simulink model "MECROKA_TWR_BLDC_02_controller_v3_1_work1"  (R2024a)
settings: Solver=FixedStepAuto  StartTime=0.0  StopTime=50  RelTol=1e-3  EnableMultiTasking=on
model workspace (MATLAB code in the model file):
  | num_pol_pairs = 7;
  | res_period = 5000;
  | res_pwm   = 2^8;
  | 
  | whl.rad = 0.045;
  | axle.length=0.18;
undefined symbols (not defined in the file): DiscIntNeverNeededParam
libraries: MecRoKa_SFunction_Library x16, simulink x3, slpidlib x1
settings Model: ExtModeTrigDuration=2  Creator=Bitsch  LastModifiedBy=Ishant
settings SolverCC: AlgebraicLoopSolver=TrustRegion  AutoInsertRateTranBlk=on
settings OptimizationCC: EnhancedBackFolding=on  PassReuseOutputArgsAs=Individual arguments  ZeroExternalMemoryAtStartup=off  ZeroInternalMemoryAtStartup=off  MaxStackSize=64  OptimizeBlockOrder=speed  DifferentSizesBufferReuse=on  EfficientTunableParamExpr=on
settings DebuggingCC: ParameterPrecisionLossMsg=none  ParameterTunabilityLossMsg=error  UnconnectedInputMsg=warning  UnconnectedOutputMsg=warning  UnconnectedLineMsg=warning
settings HardwareCC: ProdBitPerPointer=32  ProdBitPerSizeT=32  ProdBitPerPtrDiffT=32  ProdLargestAtomicInteger=Long  ProdLargestAtomicFloat=Double  ProdWordSize=32  ProdHWDeviceType=ARM Compatible->ARM Cortex
settings ModelReferenceCC: EnableRefExpFcnMdlSchedulingChecks=on
settings SFSimCC: MATLABDynamicMemAlloc=off
settings RTWCC: Description=Embedded Coder  SystemTargetFile=ert.tlc  HardwareBoard=Arduino MKR WiFi 1010  TemplateMakefile=ert_default_tmf  Toolchain=Arduino ARM  BuildConfiguration=Faster Runs  GPUComputeCapability=3.5
settings CodeAppCC: ForceParamTrailComments=on  IgnoreCustomStorageClasses=off  MaxIdLength=255  OperatorAnnotations=on  SimulinkDataObjDesc=on  SFDataObjDesc=on  InsertBlockDesc=on
settings ERTTargetCC: SupportContinuousTime=on  SupportVariableSizeSignals=on  ExtModeStaticAllocSize=8192

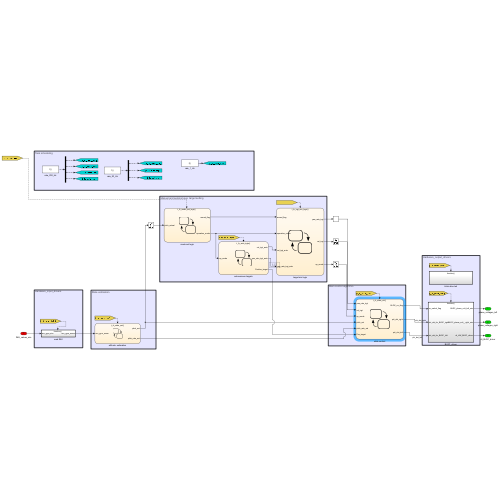
[thumbnail: Simulink's stored preview of the top-level diagram]
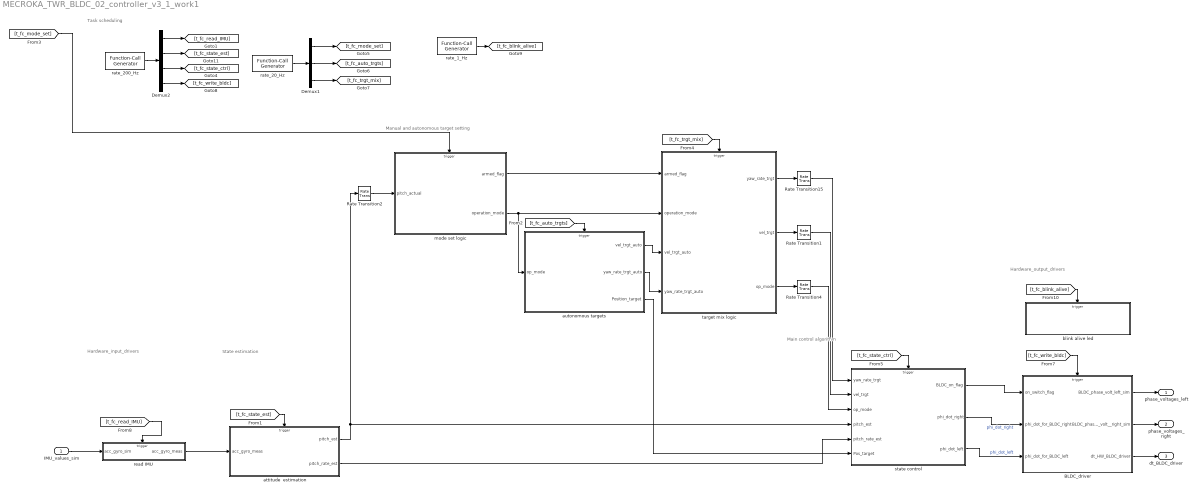
== system MECROKA_TWR_BLDC_02_controller_v3_1_work1 ==
  note: Hardware_output_drivers
  note: Main control algorithm
  note: State estimation
  note: Task scheduling
  note: Manual and autonomous target setting
  note: Hardware_input_drivers
  IMU_values_sim : Inport  OutDataTypeStr=int32  PortDimensions=6
  BLDC_driver : Subsystem  TreatAsAtomicUnit=on
  Demux1 : Demux  Outputs=3
  Demux2 : Demux
  Rate Transition{1..2,4,15} (4 alike) : RateTransition  OutPortSampleTimeOpt=Inherit  OutPortSampleTime=0.01
  attitude  estimation : Stateflow chart  TreatAsAtomicUnit=on
  autonomous targets : Stateflow chart  TreatAsAtomicUnit=on
  blink alive led : Subsystem  TreatAsAtomicUnit=on
  mode set logic : Stateflow chart  TreatAsAtomicUnit=on
  rate_1_Hz : simulink/Ports & Subsystems/Function-Call Generator  sample_time=0.5  numberOfIterations=1  DisallowWideOutput=off
  rate_200_Hz : simulink/Ports & Subsystems/Function-Call Generator  sample_time=0.005  numberOfIterations=1  DisallowWideOutput=off
  rate_20_Hz : simulink/Ports & Subsystems/Function-Call Generator  sample_time=0.05  numberOfIterations=1  DisallowWideOutput=off
  read IMU : Subsystem  TreatAsAtomicUnit=on
  state control : Stateflow chart  TreatAsAtomicUnit=on
  target mix logic : Stateflow chart  TreatAsAtomicUnit=on
  phase_voltages_left : Outport
  phase_voltages_right : Outport  Port=2
  dt_BLDC_driver : Outport  Port=3
  wires:
  autonomous targets/1(vel_trgt_auto) -> target mix logic/3(vel_trgt_auto)
  attitude  estimation/1(pitch_est) -> Rate Transition2/1, state control/4(pitch_est)
  state control/2(phi_dot_right) -> BLDC_driver/2(phi_dot_for_BLDC_right)  "phi_dot_right"
  [t_fc_trgt_mix] -> target mix logic/Trigger
  [t_fc_read_IMU] -> read IMU/Trigger
  [t_fc_state_est] -> attitude  estimation/Trigger
  Demux2/3 -> [t_fc_state_ctrl]
  Demux1/2 -> [t_fc_auto_trgts]
  Demux2/4 -> [t_fc_write_bldc]
  target mix logic/3(op_mode) -> Rate Transition4/1
  Rate Transition1/1 -> state control/2(vel_trgt)
  Demux2/1 -> [t_fc_read_IMU]
  mode set logic/1(armed_flag) -> target mix logic/1(armed_flag)
  Rate Transition15/1 -> state control/1(yaw_rate_trgt)
  Demux2/2 -> [t_fc_state_est]
  attitude  estimation/2(pitch_rate_est) -> state control/5(pitch_rate_est)
  mode set logic/2(operation_mode) -> autonomous targets/1(op_mode), target mix logic/2(operation_mode)
  IMU_values_sim/1 -> read IMU/1(acc_gyro_sim)
  [t_fc_mode_set] -> mode set logic/Trigger
  rate_200_Hz/1 -> Demux2/1
  state control/1(BLDC_on_flag) -> BLDC_driver/1(on_switch_flag)
  Rate Transition2/1 -> mode set logic/1(pitch_actual)
  [t_fc_blink_alive] -> blink alive led/Trigger
  BLDC_driver/1(BLDC_phase_volt_left_sim) -> phase_voltages_left/1
  [t_fc_auto_trgts] -> autonomous targets/Trigger
  Rate Transition4/1 -> state control/3(op_mode)
  autonomous targets/2(yaw_rate_trgt_auto) -> target mix logic/4(yaw_rate_trgt_auto)
  BLDC_driver/2(BLDC_phase_volt__right_sim) -> phase_voltages_right/1
  Demux1/3 -> [t_fc_trgt_mix]
  [t_fc_write_bldc] -> BLDC_driver/Trigger
  Demux1/1 -> [t_fc_mode_set]
  state control/3(phi_dot_left) -> BLDC_driver/3(phi_dot_for_BLDC_left)  "phi_dot_left"
  rate_20_Hz/1 -> Demux1/1
  read IMU/1(acc_gyro_meas) -> attitude  estimation/1(acc_gyro_meas)
  [t_fc_state_ctrl] -> state control/Trigger
  rate_1_Hz/1 -> [t_fc_blink_alive]
  target mix logic/1(yaw_rate_trgt) -> Rate Transition15/1
  target mix logic/2(vel_trgt) -> Rate Transition1/1
  BLDC_driver/3(dt_HW_BLDC_driver) -> dt_BLDC_driver/1
  autonomous targets/3(Position_target) -> state control/6(Pos_target)

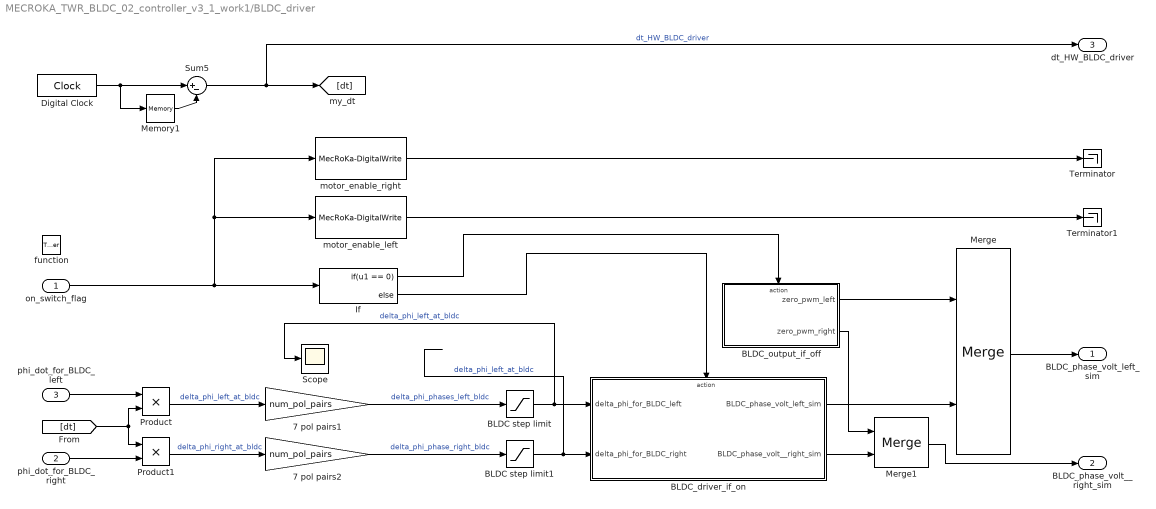
== system MECROKA_TWR_BLDC_02_controller_v3_1_work1/BLDC_driver ==
  on_switch_flag : Inport  OutDataTypeStr=boolean  PortDimensions=1
  phi_dot_for_BLDC_right : Inport  Port=2  OutDataTypeStr=double  PortDimensions=1
  phi_dot_for_BLDC_left : Inport  Port=3  OutDataTypeStr=double  PortDimensions=1
  function : TriggerPort  TriggerType=function-call  VariantControl=(inherit)
  7 pol pairs1 : Gain  Gain=num_pol_pairs
  7 pol pairs2 : Gain  Gain=num_pol_pairs
  BLDC step limit : Saturate  UpperLimit=2  LowerLimit=-2
  BLDC step limit1 : Saturate  UpperLimit=2  LowerLimit=-2
  BLDC_driver_if_on : Subsystem  TreatAsAtomicUnit=on
  BLDC_output_if_off : Subsystem  TreatAsAtomicUnit=on
  Digital Clock : DigitalClock  SampleTime=-1
  If : If  IfExpression=u1 == 0
  Memory1 : Memory  InitialCondition=-0.005  InheritSampleTime=on  LinearizeAsDelay=on
  Merge : Merge
  Merge1 : Merge
  Product : Product
  Product1 : Product
  Scope : Scope
  Sum5 : Sum  Inputs=|+-
  Terminator : Terminator
  Terminator1 : Terminator
  motor_enable_left : MecRoKa_SFunction_Library/Arduino-Blocks/Arduino-Library/MecRoKa-DigitalWrite  pinNumber=7
      settings: SourceProductName=MecRoKa_SFunction-Library
  motor_enable_right : MecRoKa_SFunction_Library/Arduino-Blocks/Arduino-Library/MecRoKa-DigitalWrite  pinNumber=6
      settings: SourceProductName=MecRoKa_SFunction-Library
  BLDC_phase_volt_left_sim : Outport  OutDataTypeStr=uint16  PortDimensions=3
  BLDC_phase_volt__right_sim : Outport  Port=2  OutDataTypeStr=uint16  PortDimensions=3
  dt_HW_BLDC_driver : Outport  Port=3
  wires:
  phi_dot_for_BLDC_right/1 -> Product1/2
  on_switch_flag/1 -> motor_enable_left/1, motor_enable_right/1, If/1
  BLDC_output_if_off/1(zero_pwm_left) -> Merge/1
  Merge/1 -> BLDC_phase_volt_left_sim/1
  If/1 -> BLDC_output_if_off/Action
  Merge1/1 -> BLDC_phase_volt__right_sim/1
  BLDC_driver_if_on/1(BLDC_phase_volt_left_sim) -> Merge/2
  If/2 -> BLDC_driver_if_on/Action
  BLDC_driver_if_on/2(BLDC_phase_volt__right_sim) -> Merge1/2
  BLDC_output_if_off/2(zero_pwm_right) -> Merge1/1
  phi_dot_for_BLDC_left/1 -> Product/1
  7 pol pairs2/1 -> BLDC step limit1/1  "delta_phi_phase_right_bldc"
  7 pol pairs1/1 -> BLDC step limit/1  "delta_phi_phases_left_bldc"
  Digital Clock/1 -> Memory1/1, Sum5/1
  Sum5/1 -> dt_HW_BLDC_driver/1, [dt]  "dt_HW_BLDC_driver"
  Memory1/1 -> Sum5/2
  [dt] -> Product1/1, Product/2
  Product/1 -> 7 pol pairs1/1  "delta_phi_left_at_bldc"
  Product1/1 -> 7 pol pairs2/1  "delta_phi_right_at_bldc"
  BLDC step limit/1 -> Scope/1, BLDC_driver_if_on/1(delta_phi_for_BLDC_left)  "delta_phi_left_at_bldc"
  BLDC step limit1/1 -> BLDC_driver_if_on/2(delta_phi_for_BLDC_right)  "delta_phi_left_at_bldc"
  motor_enable_right/1 -> Terminator/1
  motor_enable_left/1 -> Terminator1/1

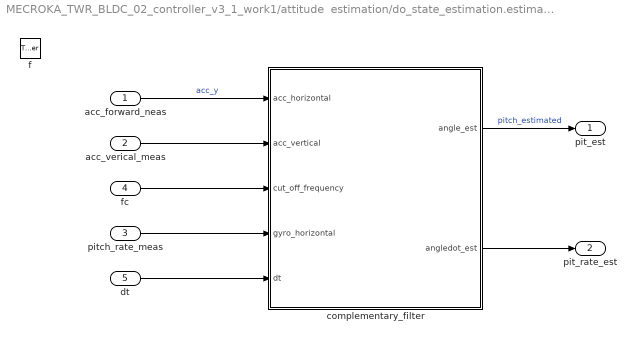
== system MECROKA_TWR_BLDC_02_controller_v3_1_work1/attitude  estimation/do_state_estimation.estimate_angulars_graph ==
  acc_forward_neas : Inport  OutDataTypeStr=double  PortDimensions=1
  acc_verical_meas : Inport  Port=2  OutDataTypeStr=double  PortDimensions=1
  pitch_rate_meas : Inport  Port=3  OutDataTypeStr=double  PortDimensions=1  LockScale=on
  fc : Inport  Port=4  OutDataTypeStr=double  PortDimensions=1
  dt : Inport  Port=5  OutDataTypeStr=double  PortDimensions=1
  f : TriggerPort  TriggerType=function-call  VariantControl=(inherit)
      settings: CopyFcn=Stateflow.SLINSF.SimulinkMan.removeBlockPreDeleteFcn  PreDeleteFcn=Stateflow.SLINSF.SimulinkMan.unsafePredeleteFcn
  complementary_filter : Subsystem
  pit_est : Outport  OutDataTypeStr=double
  pit_rate_est : Outport  Port=2  OutDataTypeStr=double
  wires:
  acc_verical_meas/1 -> complementary_filter/2(acc_vertical)
  pitch_rate_meas/1 -> complementary_filter/4(gyro_horizontal)
  acc_forward_neas/1 -> complementary_filter/1(acc_horizontal)  "acc_y"
  fc/1 -> complementary_filter/3(cut_off_frequency)
  complementary_filter/2(angledot_est) -> pit_rate_est/1
  complementary_filter/1(angle_est) -> pit_est/1  "pitch_estimated"
  dt/1 -> complementary_filter/5(dt)

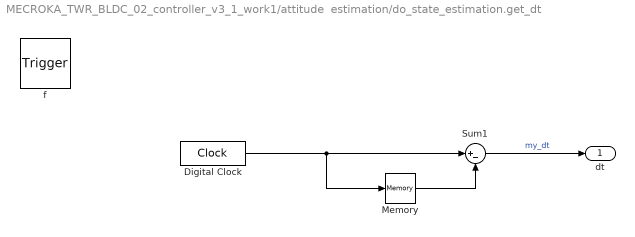
== system MECROKA_TWR_BLDC_02_controller_v3_1_work1/attitude  estimation/do_state_estimation.get_dt ==
  f : TriggerPort  TriggerType=function-call  VariantControl=(inherit)
      settings: CopyFcn=Stateflow.SLINSF.SimulinkMan.removeBlockPreDeleteFcn  PreDeleteFcn=Stateflow.SLINSF.SimulinkMan.unsafePredeleteFcn
  Digital Clock : DigitalClock  SampleTime=-1
  Memory : Memory  InitialCondition=-0.005  InheritSampleTime=on  LinearizeAsDelay=on
  Sum1 : Sum  Inputs=|+-
  dt : Outport
  wires:
  Sum1/1 -> dt/1  "my_dt"
  Digital Clock/1 -> Memory/1, Sum1/1
  Memory/1 -> Sum1/2

== system MECROKA_TWR_BLDC_02_controller_v3_1_work1/blink alive led ==
  function : TriggerPort  TriggerType=function-call  VariantControl=(inherit)
  MecRoKa-TogglePin : MecRoKa_SFunction_Library/Arduino-Blocks/Arduino-Library/MecRoKa-TogglePin  pinNumber=13
      settings: SourceProductName=MecRoKa_SFunction-Library

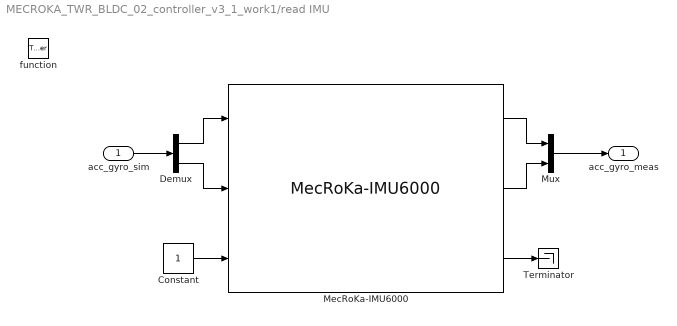
== system MECROKA_TWR_BLDC_02_controller_v3_1_work1/read IMU ==
  acc_gyro_sim : Inport  OutDataTypeStr=int32  PortDimensions=6
  function : TriggerPort  TriggerType=function-call  VariantControl=(inherit)
  Constant : Constant  OutDataTypeStr=int32
  Demux : Demux  Outputs=2
  MecRoKa-IMU6000 : MecRoKa_SFunction_Library/Arduino-Blocks/Sensor-Library/MecRoKa-IMU6000  selectWire=0
      settings: SourceProductName=MecRoKa_SFunction-Library
  Mux : Mux  Inputs=2
  Terminator : Terminator
  acc_gyro_meas : Outport  OutDataTypeStr=int32  PortDimensions=6
  wires:
  acc_gyro_sim/1 -> Demux/1
  Mux/1 -> acc_gyro_meas/1
  Demux/1 -> MecRoKa-IMU6000/1
  Demux/2 -> MecRoKa-IMU6000/2
  MecRoKa-IMU6000/1 -> Mux/1
  MecRoKa-IMU6000/2 -> Mux/2
  MecRoKa-IMU6000/3 -> Terminator/1
  Constant/1 -> MecRoKa-IMU6000/3

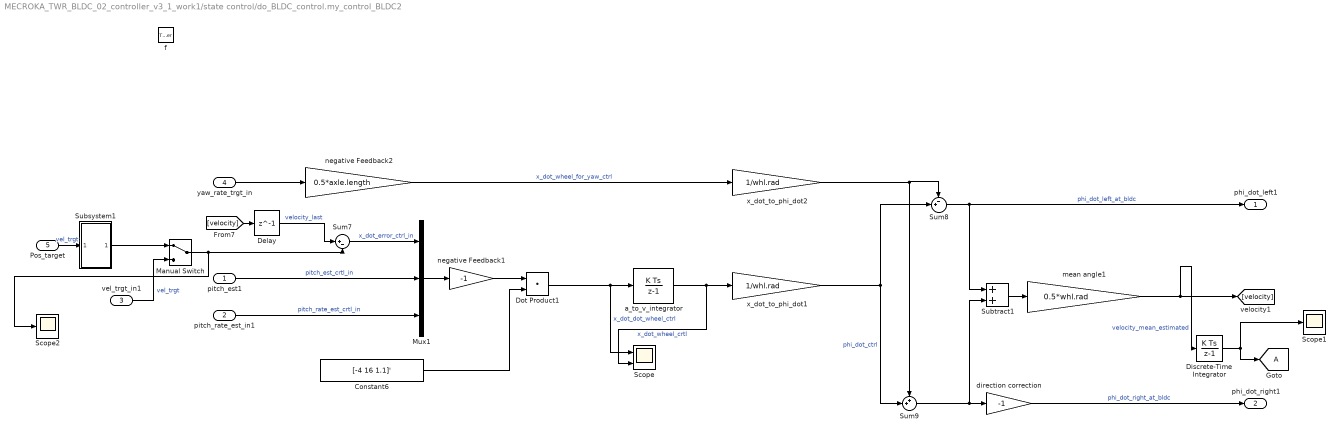
== system MECROKA_TWR_BLDC_02_controller_v3_1_work1/state control/do_BLDC_control.my_control_BLDC2 ==
  pitch_est1 : Inport  OutDataTypeStr=double  PortDimensions=1
  pitch_rate_est_in1 : Inport  Port=2  OutDataTypeStr=double  PortDimensions=1
  vel_trgt_in1 : Inport  Port=3  OutDataTypeStr=double  PortDimensions=1
  yaw_rate_trgt_in : Inport  Port=4  OutDataTypeStr=double  PortDimensions=1
  Pos_target : Inport  Port=5  OutDataTypeStr=double  PortDimensions=1
  f : TriggerPort  TriggerType=function-call  VariantControl=(inherit)
      settings: CopyFcn=Stateflow.SLINSF.SimulinkMan.removeBlockPreDeleteFcn  PreDeleteFcn=Stateflow.SLINSF.SimulinkMan.unsafePredeleteFcn
  Constant6 : Constant  Value=[-4 16 1.1]'  OutDataTypeStr=double
  Delay : Delay  DelayLength=1  InitialCondition=0
  Discrete-Time Integrator : DiscreteIntegrator  SampleTime=-1  ICPrevOutput=DiscIntNeverNeededParam  ICPrevScaledInput=DiscIntNeverNeededParam
  Dot Product1 : DotProduct  OutDataTypeStr=Inherit: Inherit via internal rule
  Goto : Goto  TagVisibility=global
  Manual Switch : ManualSwitch
  Mux1 : Mux  Inputs=3
  Scope : Scope  NumInputPorts=2
  Scope1 : Scope
  Scope2 : Scope
  Subsystem1 : Subsystem
  Subtract1 : Sum
  Sum7 : Sum  Inputs=|+-
  Sum8 : Sum  Inputs=-+|
  Sum9 : Sum  Inputs=++|
  a_to_v_integrator : DiscreteIntegrator  SampleTime=-1  LimitOutput=on  UpperSaturationLimit=2  LowerSaturationLimit=-5  ICPrevOutput=DiscIntNeverNeededParam  ICPrevScaledInput=DiscIntNeverNeededParam
  direction correction : Gain  Gain=-1
  mean angle1 : Gain  Gain=0.5*whl.rad  OutDataTypeStr=double
  negative Feedback1 : Gain  Gain=-1
  negative Feedback2 : Gain  Gain=0.5*axle.length
  x_dot_to_phi_dot1 : Gain  Gain=1/whl.rad
  x_dot_to_phi_dot2 : Gain  Gain=1/whl.rad
  phi_dot_left1 : Outport  OutDataTypeStr=double  PortDimensions=1
  phi_dot_right1 : Outport  Port=2  OutDataTypeStr=double  PortDimensions=1
  wires:
  Mux1/1 -> negative Feedback1/1
  negative Feedback1/1 -> Dot Product1/1
  Sum7/1 -> Mux1/1  "x_dot_error_ctrl_in"
  Constant6/1 -> Dot Product1/2
  yaw_rate_trgt_in/1 -> negative Feedback2/1
  x_dot_to_phi_dot2/1 -> Sum9/1, Sum8/1
  [velocity] -> Delay/1
  vel_trgt_in1/1 -> Manual Switch/2  "vel_trgt"
  pitch_est1/1 -> Mux1/2  "pitch_est_crtl_in"
  pitch_rate_est_in1/1 -> Mux1/3  "pitch_rate_est_crtl_in"
  Dot Product1/1 -> Scope/1, a_to_v_integrator/1  "x_dot_dot_wheel_ctrl"
  x_dot_to_phi_dot1/1 -> Sum9/2, Sum8/2  "phi_dot_ctrl"
  Sum9/1 -> Subtract1/2, direction correction/1
  Subtract1/1 -> mean angle1/1
  Delay/1 -> Sum7/1  "velocity_last"
  Sum8/1 -> Subtract1/1, phi_dot_left1/1  "phi_dot_left_at_bldc"
  direction correction/1 -> phi_dot_right1/1  "phi_dot_right_at_bldc"
  a_to_v_integrator/1 -> Scope/2, x_dot_to_phi_dot1/1  "x_dot_wheel_crtl"
  negative Feedback2/1 -> x_dot_to_phi_dot2/1  "x_dot_wheel_for_yaw_ctrl"
  mean angle1/1 -> Discrete-Time Integrator/1, [velocity]  "velocity_mean_estimated"
  Discrete-Time Integrator/1 -> Goto/1, Scope1/1
  Subsystem1/1(Output) -> Manual Switch/1
  Manual Switch/1 -> Scope2/1, Sum7/2
  Pos_target/1 -> Subsystem1/1(Input)  "vel_trgt"

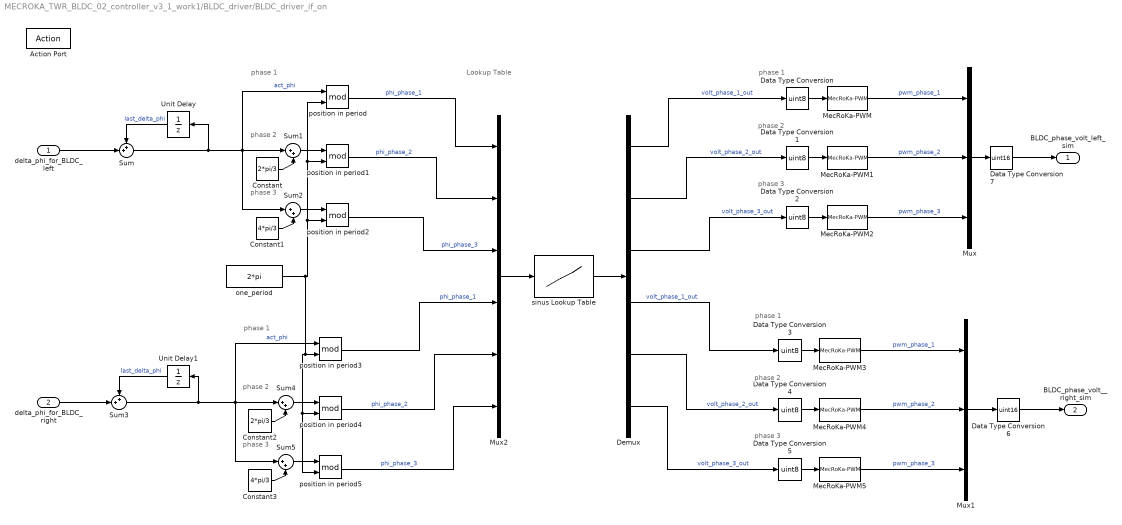
== system MECROKA_TWR_BLDC_02_controller_v3_1_work1/BLDC_driver/BLDC_driver_if_on ==
  note: Lookup Table
  note: phase 3
  note: phase 2
  note: phase 1
  note: phase 3
  note: phase 2
  note: phase 1
  note: phase 1
  note: phase 2
  note: phase 3
  note: phase 3
  note: phase 1
  note: phase 2
  delta_phi_for_BLDC_left : Inport  OutDataTypeStr=double  PortDimensions=1
  delta_phi_for_BLDC_right : Inport  Port=2  OutDataTypeStr=double  PortDimensions=1
  Action Port : ActionPort  ActionPortLabel=else
  Constant : Constant  Value=2*pi/3
  Constant1 : Constant  Value=4*pi/3
  Constant2 : Constant  Value=2*pi/3
  Constant3 : Constant  Value=4*pi/3
  Data Type Conversion{,1..5} (6 alike) : DataTypeConversion  OutDataTypeStr=uint8  SaturateOnIntegerOverflow=off  RndMeth=Floor
  Data Type Conversion6 : DataTypeConversion  OutDataTypeStr=uint16  SaturateOnIntegerOverflow=off  RndMeth=Floor
  Data Type Conversion7 : DataTypeConversion  OutDataTypeStr=uint16  SaturateOnIntegerOverflow=off  RndMeth=Floor
  Demux : Demux  Outputs=6
  MecRoKa-PWM : MecRoKa_SFunction_Library/Arduino-Blocks/Arduino-Library/MecRoKa-PWM  pinNumber=0
      settings: SourceProductName=MecRoKa_SFunction-Library
  MecRoKa-PWM1 : MecRoKa_SFunction_Library/Arduino-Blocks/Arduino-Library/MecRoKa-PWM  pinNumber=1
      settings: SourceProductName=MecRoKa_SFunction-Library
  MecRoKa-PWM2 : MecRoKa_SFunction_Library/Arduino-Blocks/Arduino-Library/MecRoKa-PWM  pinNumber=2
      settings: SourceProductName=MecRoKa_SFunction-Library
  MecRoKa-PWM3 : MecRoKa_SFunction_Library/Arduino-Blocks/Arduino-Library/MecRoKa-PWM  pinNumber=3
      settings: SourceProductName=MecRoKa_SFunction-Library
  MecRoKa-PWM4 : MecRoKa_SFunction_Library/Arduino-Blocks/Arduino-Library/MecRoKa-PWM  pinNumber=4
      settings: SourceProductName=MecRoKa_SFunction-Library
  MecRoKa-PWM5 : MecRoKa_SFunction_Library/Arduino-Blocks/Arduino-Library/MecRoKa-PWM  pinNumber=5
      settings: SourceProductName=MecRoKa_SFunction-Library
  Mux : Mux  Inputs=3
  Mux1 : Mux  Inputs=3
  Mux2 : Mux  Inputs=6
  Sum : Sum  Inputs=++|
  Sum{1..2,4..5} (4 alike) : Sum  Inputs=|++
  Sum3 : Sum  Inputs=++|
  Unit Delay : UnitDelay  SampleTime=-1  HasFrameUpgradeWarning=on
  Unit Delay1 : UnitDelay  SampleTime=-1  HasFrameUpgradeWarning=on
  one_period : Constant  Value=2*pi
  position in period{,1..5} (6 alike) : Math  Operator=mod  SignedPower=on
  sinus Lookup Table : Lookup_n-D  NumberOfTableDimensions=1  BreakpointsSpecification=Even spacing  BreakpointsForDimension1=[0:0.25:2*pi]  BreakpointsForDimension2=[0:0.25:2*pi]  BreakpointsForDimension3=[0:0.25:2*pi]  BreakpointsForDimension1FirstPoint=0  BreakpointsForDimension1Spacing=2*pi/res_period  BreakpointsForDimension2Spacing=0.25  BreakpointsForDimension3Spacing=0.25  BeginIndexSearchUsingPreviousIndexResult=on  Table=(res_pwm/2-1)*sin([0:2*pi/res_period:2*pi])+(res_pwm/2-1)  InterpMethod=Nearest  ExtrapMethod=Cubic spline  InternalRulePriority=Speed  OutDataTypeStr=uint16  RndMeth=Simplest
  BLDC_phase_volt_left_sim : Outport  OutDataTypeStr=uint16  PortDimensions=3
  BLDC_phase_volt__right_sim : Outport  Port=2  OutDataTypeStr=uint16  PortDimensions=3
  wires:
  Demux/1 -> Data Type Conversion/1  "volt_phase_1_out"
  Unit Delay/1 -> Sum/1  "last_delta_phi"
  Sum/1 -> position in period/1, Sum2/1, Sum1/1, Unit Delay/1  "act_phi"
  Sum1/1 -> position in period1/1
  Sum2/1 -> position in period2/1
  Constant/1 -> Sum1/2
  position in period1/1 -> Mux2/2  "phi_phase_2"
  position in period2/1 -> Mux2/3  "phi_phase_3"
  Demux/2 -> Data Type Conversion1/1  "volt_phase_2_out"
  Demux/3 -> Data Type Conversion2/1  "volt_phase_3_out"
  Constant1/1 -> Sum2/2
  position in period/1 -> Mux2/1  "phi_phase_1"
  Mux/1 -> Data Type Conversion7/1
  Data Type Conversion/1 -> MecRoKa-PWM/1
  Data Type Conversion1/1 -> MecRoKa-PWM1/1
  Data Type Conversion2/1 -> MecRoKa-PWM2/1
  MecRoKa-PWM/1 -> Mux/1  "pwm_phase_1"
  MecRoKa-PWM1/1 -> Mux/2  "pwm_phase_2"
  MecRoKa-PWM2/1 -> Mux/3  "pwm_phase_3"
  delta_phi_for_BLDC_left/1 -> Sum/2
  one_period/1 -> position in period5/2, position in period4/2, position in period3/2, position in period/2, position in period1/2, position in period2/2
  Unit Delay1/1 -> Sum3/1  "last_delta_phi"
  Sum3/1 -> position in period3/1, Sum5/1, Sum4/1, Unit Delay1/1  "act_phi"
  Sum4/1 -> position in period4/1
  Sum5/1 -> position in period5/1
  Constant2/1 -> Sum4/2
  position in period4/1 -> Mux2/5  "phi_phase_2"
  position in period5/1 -> Mux2/6  "phi_phase_3"
  Constant3/1 -> Sum5/2
  position in period3/1 -> Mux2/4  "phi_phase_1"
  Mux1/1 -> Data Type Conversion6/1
  Data Type Conversion3/1 -> MecRoKa-PWM3/1
  Data Type Conversion4/1 -> MecRoKa-PWM4/1
  Data Type Conversion5/1 -> MecRoKa-PWM5/1
  MecRoKa-PWM3/1 -> Mux1/1  "pwm_phase_1"
  MecRoKa-PWM4/1 -> Mux1/2  "pwm_phase_2"
  MecRoKa-PWM5/1 -> Mux1/3  "pwm_phase_3"
  Demux/4 -> Data Type Conversion3/1  "volt_phase_1_out"
  Demux/5 -> Data Type Conversion4/1  "volt_phase_2_out"
  Demux/6 -> Data Type Conversion5/1  "volt_phase_3_out"
  delta_phi_for_BLDC_right/1 -> Sum3/2
  Data Type Conversion7/1 -> BLDC_phase_volt_left_sim/1
  Data Type Conversion6/1 -> BLDC_phase_volt__right_sim/1
  Mux2/1 -> sinus Lookup Table/1
  sinus Lookup Table/1 -> Demux/1

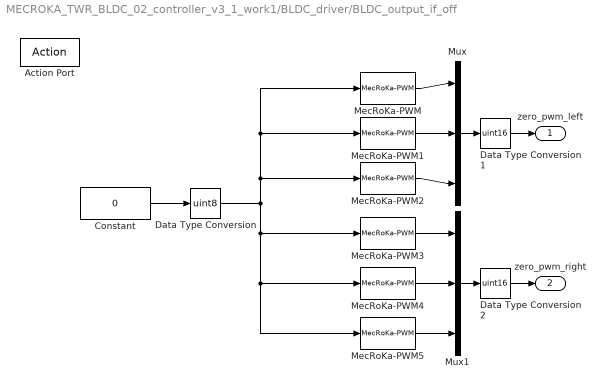
== system MECROKA_TWR_BLDC_02_controller_v3_1_work1/BLDC_driver/BLDC_output_if_off ==
  Action Port : ActionPort  ActionPortLabel=if(u1 == 0)
  Constant : Constant  Value=0  OutDataTypeStr=uint16
  Data Type Conversion : DataTypeConversion  OutDataTypeStr=uint8  SaturateOnIntegerOverflow=off  RndMeth=Floor
  Data Type Conversion1 : DataTypeConversion  OutDataTypeStr=uint16  SaturateOnIntegerOverflow=off  RndMeth=Floor
  Data Type Conversion2 : DataTypeConversion  OutDataTypeStr=uint16  SaturateOnIntegerOverflow=off  RndMeth=Floor
  MecRoKa-PWM : MecRoKa_SFunction_Library/Arduino-Blocks/Arduino-Library/MecRoKa-PWM  pinNumber=0
      settings: SourceProductName=MecRoKa_SFunction-Library
  MecRoKa-PWM1 : MecRoKa_SFunction_Library/Arduino-Blocks/Arduino-Library/MecRoKa-PWM  pinNumber=1
      settings: SourceProductName=MecRoKa_SFunction-Library
  MecRoKa-PWM2 : MecRoKa_SFunction_Library/Arduino-Blocks/Arduino-Library/MecRoKa-PWM  pinNumber=2
      settings: SourceProductName=MecRoKa_SFunction-Library
  MecRoKa-PWM3 : MecRoKa_SFunction_Library/Arduino-Blocks/Arduino-Library/MecRoKa-PWM  pinNumber=3
      settings: SourceProductName=MecRoKa_SFunction-Library
  MecRoKa-PWM4 : MecRoKa_SFunction_Library/Arduino-Blocks/Arduino-Library/MecRoKa-PWM  pinNumber=4
      settings: SourceProductName=MecRoKa_SFunction-Library
  MecRoKa-PWM5 : MecRoKa_SFunction_Library/Arduino-Blocks/Arduino-Library/MecRoKa-PWM  pinNumber=5
      settings: SourceProductName=MecRoKa_SFunction-Library
  Mux : Mux  Inputs=3
  Mux1 : Mux  Inputs=3
  zero_pwm_left : Outport
  zero_pwm_right : Outport  Port=2
  wires:
  Constant/1 -> Data Type Conversion/1
  Data Type Conversion/1 -> MecRoKa-PWM5/1, MecRoKa-PWM4/1, MecRoKa-PWM3/1, MecRoKa-PWM1/1, MecRoKa-PWM/1, MecRoKa-PWM2/1
  MecRoKa-PWM/1 -> Mux/1
  MecRoKa-PWM1/1 -> Mux/2
  MecRoKa-PWM2/1 -> Mux/3
  MecRoKa-PWM3/1 -> Mux1/1
  MecRoKa-PWM4/1 -> Mux1/2
  MecRoKa-PWM5/1 -> Mux1/3
  Mux1/1 -> Data Type Conversion2/1
  Mux/1 -> Data Type Conversion1/1
  Data Type Conversion1/1 -> zero_pwm_left/1
  Data Type Conversion2/1 -> zero_pwm_right/1

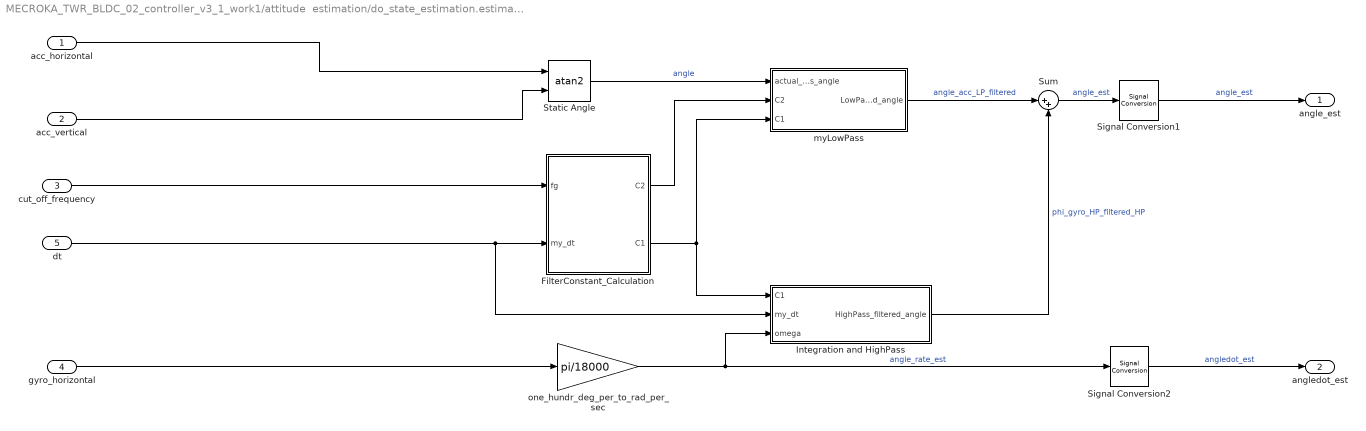
== system MECROKA_TWR_BLDC_02_controller_v3_1_work1/attitude  estimation/do_state_estimation.estimate_angulars_graph/complementary_filter ==
  acc_horizontal : Inport
  acc_vertical : Inport  Port=2
  cut_off_frequency : Inport  Port=3
  gyro_horizontal : Inport  Port=4
  dt : Inport  Port=5
  FilterConstant_Calculation : Subsystem
  Integration and HighPass : Subsystem
  Signal Conversion1 : SignalConversion  OverrideOpt=off
  Signal Conversion2 : SignalConversion  OverrideOpt=off
  Static Angle : Trigonometry  Operator=atan2  OutputSignalType=real
  Sum : Sum  Inputs=|++
  myLowPass : Subsystem  TreatAsAtomicUnit=on
  one_hundr_deg_per_to_rad_per_sec : Gain  Gain=pi/18000
  angle_est : Outport  PortDimensions=1
  angledot_est : Outport  Port=2  PortDimensions=1
  wires:
  FilterConstant_Calculation/2(C1) -> myLowPass/3(C1), Integration and HighPass/1(C1)
  myLowPass/1(LowPass_filtered_angle) -> Sum/1  "angle_acc_LP_filtered"
  cut_off_frequency/1 -> FilterConstant_Calculation/1(fg)
  one_hundr_deg_per_to_rad_per_sec/1 -> Signal Conversion2/1, Integration and HighPass/3(omega)  "angle_rate_est"
  Static Angle/1 -> myLowPass/1(actual_meas_angle)  "angle"
  FilterConstant_Calculation/1(C2) -> myLowPass/2(C2)
  Sum/1 -> Signal Conversion1/1  "angle_est"
  Integration and HighPass/1(HighPass_filtered_angle) -> Sum/2  "phi_gyro_HP_filtered_HP"
  gyro_horizontal/1 -> one_hundr_deg_per_to_rad_per_sec/1
  Signal Conversion2/1 -> angledot_est/1  "angledot_est"
  acc_vertical/1 -> Static Angle/2
  Signal Conversion1/1 -> angle_est/1  "angle_est"
  acc_horizontal/1 -> Static Angle/1
  dt/1 -> Integration and HighPass/2(my_dt), FilterConstant_Calculation/2(my_dt)

== system MECROKA_TWR_BLDC_02_controller_v3_1_work1/state control/do_BLDC_control.my_control_BLDC2/Subsystem1 ==
  Input : Inport
  Discrete PID Controller : slpidlib/PID Controller  Controller=PID  Form=Parallel  TimeDomain=Discrete-time  UseExternalTs=off  SampleTime=-1  IntegratorMethod=Forward Euler  FilterMethod=Forward Euler  ControllerParametersSource=internal  P=0.37  I=0.1  UseKiTs=off  D=0.01  UseExternalDerivativeSource=off  N=150  UseFilter=on  TunerSelectOption=Frequency Response Based  InitialConditionSource=internal  InitialConditionForIntegrator=0  InitialConditionForFilter=0  DifferentiatorICPrevScaledInput=0  ExternalReset=none  TrackingMode=off  Kt=1  LimitOutput=off  SatLimitsSource=internal  UpperSaturationLimit=inf  LowerSaturationLimit=-inf  LinearizeAsGain=off  AntiWindupMode=none  Kb=1  LimitIntegrator=off  UpperIntegratorSaturationLimit=inf  LowerIntegratorSaturationLimit=-inf  POutMin=[]  POutMax=[]  IOutMin=[]  IOutMax=[]  DOutMin=[]  DOutMax=[]  NOutMin=[]  NOutMax=[]  SumOutMin=[]  SumOutMax=[]  SaturationOutMin=[]  SaturationOutMax=[]  PParamMin=[]  PParamMax=[]  IParamMin=[]  IParamMax=[]  DParamMin=[]  DParamMax=[]  NParamMin=[]  NParamMax=[]  KbParamMin=[]  KbParamMax=[]  KtParamMin=[]  KtParamMax=[]  KbOutMin=[]  KbOutMax=[]  KtOutMin=[]  KtOutMax=[]  IntegratorOutMin=[]  IntegratorOutMax=[]  FilterOutMin=[]  FilterOutMax=[]  SumI1OutMin=[]  SumI1OutMax=[]  SumI2OutMin=[]  SumI2OutMax=[]  SumI3OutMin=[]  SumI3OutMax=[]  SumI4OutMin=[]  SumI4OutMax=[]  SumDOutMin=[]  SumDOutMax=[]  DifferentiatorOutMin=[]  DifferentiatorOutMax=[]  FilterDiffOutCoefMin=[]  FilterDiffOutCoefMax=[]  ReciprocalOutMin=[]  ReciprocalOutMax=[]  SumDenOutMin=[]  SumDenOutMax=[]  SumNumOutMin=[]  SumNumOutMax=[]  DivideOutMin=[]  DivideOutMax=[]  UdiffTsProdOutMin=[]  UdiffTsProdOutMax=[]  NTsProdOutMin=[]  NTsProdOutMax=[]  UintegralTsProdOutMin=[]  UintegralTsProdOutMax=[]  UngainTsProdOutMin=[]  UngainTsProdOutMax=[]  ClampingZeroOutDataTypeStr=Inherit: Inherit via back propagation  ClampingZeroOutMin=[]  ClampingZeroOutMax=[]  FilterDenConstantOutDataTypeStr=Inherit: Inherit via back propagation  FilterDenConstantOutMin=[]  FilterDenConstantOutMax=[]  PCopyOutDataTypeStr=Inherit: Inherit via back propagation  PCopyOutMin=[]  PCopyOutMax=[]  NCopyOutDataTypeStr=Inherit: Inherit via back propagation  NCopyOutMin=[]  NCopyOutMax=[]  IntegratorContinuousStateAttributes=''  IntegratorStateMustResolveToSignalObject=off  IntegratorRTWStateStorageClass=Auto  FilterContinuousStateAttributes=''  FilterStateMustResolveToSignalObject=off  FilterRTWStateStorageClass=Auto  ParallelPVariant=InternalParameters  IdealPVariant=Disabled  IVariant=InternalParameters  DVariant=InternalParameters  IntegratorVariant=Discrete  SatVariant=Disabled  AWVariant=Passthrough  PCopyVariant=Disabled  TRVariant=Disabled  FdbkBlocksVariant=Forward  IdealPFdbkVariant=Disabled  SatFdbkVariant=Disabled  DerivativeFilterVariant=ForwardEulerFilter  NVariant=InternalParameters  NCopyVariant=Disabled  FilterICVariant=InternalICsFilter  IntegratorICVariant=InternalICs  ExternalResetVariant=Disabled  TRSumVariant=Passthrough  SumFdbkVariant=Disabled  SumVariant=Sum_PID  TsampFilterVariant=InternalTs  TsampNgainVariant=Passthrough  TsampIntegralVariant=Disabled_SignalSpec  ExternalSaturationOutDataTypeStr=Inherit: Same as second input  DerivativeSourceVariant=ErrorSignal
      settings: LibrarySourceBlock=simulink/Discrete/Discrete PID Controller
  Gain : Gain
  Subsystem : Subsystem
  Output : Outport
  wires:
  Gain/1 -> Output/1
  Input/1 -> Subsystem/1(Input)
  Discrete PID Controller/1 -> Gain/1
  Subsystem/1(Output) -> Discrete PID Controller/1

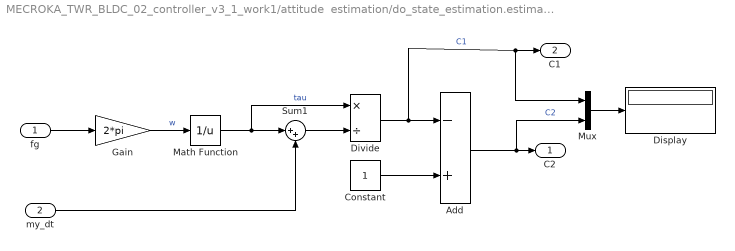
== system MECROKA_TWR_BLDC_02_controller_v3_1_work1/attitude  estimation/do_state_estimation.estimate_angulars_graph/complementary_filter/FilterConstant_Calculation ==
  fg : Inport
  my_dt : Inport  Port=2
  Add : Sum  Inputs=-+
  Constant : Constant
  Display : Display
      settings: Decimation=3
  Divide : Product  Inputs=*/
  Gain : Gain  Gain=2*pi
  Math Function : Math  Operator=reciprocal  SignedPower=on
  Mux : Mux  Inputs=2
  Sum1 : Sum  Inputs=|++
  C2 : Outport
  C1 : Outport  Port=2
  wires:
  Math Function/1 -> Divide/1, Sum1/1  "tau"
  Gain/1 -> Math Function/1  "w"
  Sum1/1 -> Divide/2
  fg/1 -> Gain/1
  my_dt/1 -> Sum1/2
  Divide/1 -> Mux/1, C1/1, Add/1  "C1"
  Constant/1 -> Add/2
  Add/1 -> Mux/2, C2/1  "C2"
  Mux/1 -> Display/1

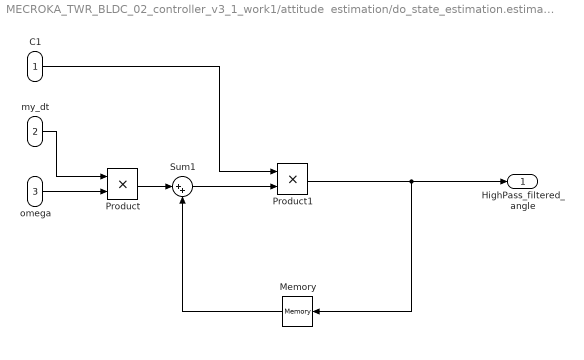
== system MECROKA_TWR_BLDC_02_controller_v3_1_work1/attitude  estimation/do_state_estimation.estimate_angulars_graph/complementary_filter/Integration and HighPass ==
  C1 : Inport
  my_dt : Inport  Port=2
  omega : Inport  Port=3
  Memory : Memory  InheritSampleTime=on
  Product : Product  RndMeth=Zero
  Product1 : Product  RndMeth=Zero
  Sum1 : Sum  Inputs=|++
  HighPass_filtered_angle : Outport
  wires:
  Memory/1 -> Sum1/2
  Product1/1 -> Memory/1, HighPass_filtered_angle/1
  Product/1 -> Sum1/1
  omega/1 -> Product/2
  my_dt/1 -> Product/1
  Sum1/1 -> Product1/2
  C1/1 -> Product1/1

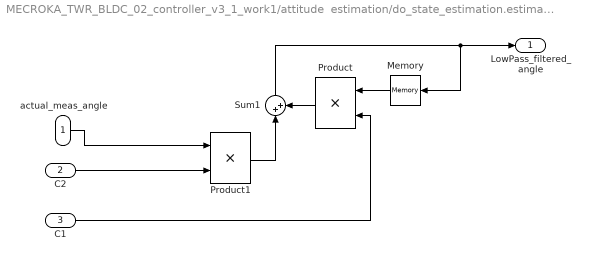
== system MECROKA_TWR_BLDC_02_controller_v3_1_work1/attitude  estimation/do_state_estimation.estimate_angulars_graph/complementary_filter/myLowPass ==
  actual_meas_angle : Inport  OutDataTypeStr=double
  C2 : Inport  Port=2
  C1 : Inport  Port=3
  Memory : Memory  InitialCondition=0*pi/180  InheritSampleTime=on
  Product : Product  RndMeth=Zero
  Product1 : Product  RndMeth=Zero
  Sum1 : Sum  Inputs=|++
  LowPass_filtered_angle : Outport
  wires:
  actual_meas_angle/1 -> Product1/1
  Sum1/1 -> Memory/1, LowPass_filtered_angle/1
  Product/1 -> Sum1/2
  Product1/1 -> Sum1/1
  C1/1 -> Product/2
  Memory/1 -> Product/1
  C2/1 -> Product1/2

== system MECROKA_TWR_BLDC_02_controller_v3_1_work1/state control/do_BLDC_control.my_control_BLDC2/Subsystem1/Subsystem ==
  Input : Inport
  From : From  TagVisibility=global
  Sum : Sum  Inputs=-+
  Output : Outport
  wires:
  Sum/1 -> Output/1
  From/1 -> Sum/1
  Input/1 -> Sum/2

== stateflow chart MECROKA_TWR_BLDC_02_controller_v3_1_work1/state control ==
  state system_off
    en, du: phi_dot_left   = double(0.0);
    en, du: phi_dot_right = double(0.0);
    en, du: BLDC_on_flag = false;
  state do_BLDC_control
    en, du: BLDC_on_flag = true;
    en, du : [phi_dot_left, phi_dot_right]=my_control_BLDC2(pitch_est, pitch_rate_est, vel_trgt, yaw_rate_trgt,Pos_target);
    state [phi_dot_left1,phi_dot_right1] = my_control_BLDC2(pitch_est1,pitch_rate_est_in1,vel_trgt_in1,yaw_rate_trgt_in,Pos_target) [function]
  (default) -> system_off
  system_off -> do_BLDC_control : [op_mode ~= 0 ]
  do_BLDC_control -> system_off : [op_mode == 0 ]
  data: pitch_est1 function_input double size=1; pitch_rate_est_in1 function_input double size=1; vel_trgt_in1 function_input double size=1; yaw_rate_trgt_in function_input double size=1; phi_dot_left1 function_output double size=1; phi_dot_right1 function_output double size=1; Pos_target function_input double size=1; BLDC_on_flag output boolean; yaw_rate_trgt input double size=1; vel_trgt input double size=1; op_mode input uint8; pitch_est input double size=1; pitch_rate_est input double size=1; phi_dot_right output; phi_dot_left output; Pos_target input double size=1
  events: t_fc_state_ctrl input FUNCTION_CALL_EVENT

== stateflow chart MECROKA_TWR_BLDC_02_controller_v3_1_work1/target mix logic ==
  state disarmed
    en, du: op_mode = uint8(0);
    en, du: vel_trgt = 0;
    en, du: yaw_rate_trgt  = 0;
  state armed
    en, du: op_mode = operation_mode;
    en, du: yaw_rate_trgt  = yaw_rate_trgt_auto;
    state autonomous
      en, du: vel_trgt   = vel_trgt_auto;
    (default) -> (junction 18)
    (junction 18) -> autonomous
  (default) -> (junction 15)
  (junction 15) -> armed [order 1] : [armed_flag == true]
  (junction 15) -> disarmed [order 2]
  disarmed -> armed : [armed_flag == true]
  armed -> disarmed : [armed_flag == false]
  data: yaw_rate_trgt output double size=1; vel_trgt output double size=1; armed_flag input boolean size=1; operation_mode input uint8 size=1; vel_trgt_auto input double size=1; yaw_rate_trgt_auto input double size=1; op_mode output uint8
  events: t_fc_trgt_mix_logic input FUNCTION_CALL_EVENT

== stateflow chart MECROKA_TWR_BLDC_02_controller_v3_1_work1/attitude  estimation ==
  state do_state_estimation
    en: cut_off_freq = 1.;
    en: step_size = get_dt();
    en: [pitch_est, pitch_rate_est] = estimate_angulars_script(double(acc_gyro_meas(2)), double(acc_gyro_meas(3)), double(acc_gyro_meas(4)),cut_off_freq, step_size );
    state dt = get_dt [function]
    state [pit_est, pit_rate_est] = estimate_angulars_graph(acc_forward_neas, acc_verical_meas, pitch_rate_meas, fc, dt) [function]
  (default) -> do_state_estimation
  do_state_estimation -> do_state_estimation
  data: dt function_output; acc_forward_neas function_input double size=1; acc_verical_meas function_input double size=1; pit_est function_output double; pitch_rate_meas function_input double size=1; pit_rate_est function_output double; fc function_input double size=1; dt function_input double size=1; acc_forward_meas function_input; acc_vertical_meas function_input; pitch_rate_meas function_input; pit_est function_output; pit_rate_est function_output; fc function_input; dt function_input; pitch_est output double size=1; pitch_rate_est output double size=1; acc_gyro_meas input int32 size=6; cut_off_freq local; step_size local double size=1
  events: t_fc_state_est input FUNCTION_CALL_EVENT
  function [pit_est, pit_rate_est] = estimate_angulars_script(acc_forward_meas, acc_vertical_meas, pitch_rate_meas, fc, dt ):
    | function [pit_est, pit_rate_est] = estimate_angulars_script(acc_forward_meas, acc_vertical_meas, pitch_rate_meas, fc, dt )
    | % created by GBi 14.05.2020
    | % complementary filter combines high (HP) and low pass (LP) filter 
    | % signals with the same cutoff-frequency fc
    | %
    | % transfer function for LP: 1/(tau*s+1)
    | % transfer function for HP: tau*s/(tau*s+1)
    | % combining a HP with an integration (multiply with 1/s) yields: tau/(tau*s+1)
    | %
    | % first order approximation with time step size dt yields
    | % for LP:               new_value = C*old_value +(1-C)*actual_value
    | % for HP + integration: new_value = C*(old_value + delta_t*actual_value)
    | % with constant C = tau/(tau+dt)
    | %
    | % with cutoff angular frequency omega_c=1/tau and omega_c=2*pi*fc
    | % tau = 1./(2*pi*fc)
    | %
    | % complementry filter here combines LP filtered pitch estimation
    | % based on accelerometer data and integrated HP filtered pitch estimation
    | % based on gyro data
    | %
    | %----------------------------------------------------------------------------
    | persistent tau C pitch_from_acc_LP_filtered pitch_from_gyro_HP_filtered
    | if isempty(tau);
    |     tau = 1./ (2*pi*fc);
    |     C = tau/(tau+dt);
    |     pitch_from_acc_LP_filtered = 0.0;
    |     pitch_from_gyro_HP_filtered = 0.0;
    | end 
    | pitch_from_acc = atan2(acc_forward_meas, acc_vertical_meas);
    | pit_rate_est = pitch_rate_meas*pi/18000; %result in [rad/s]
    | pitch_from_acc_LP_filtered  = C*pitch_from_acc_LP_filtered +(1-C)*pitch_from_acc;
    | pitch_from_gyro_HP_filtered = C*(pitch_from_gyro_HP_filtered+pit_rate_est*dt);
    | pit_est = pitch_from_acc_LP_filtered + pitch_from_gyro_HP_filtered; %result in [rad]

== stateflow chart MECROKA_TWR_BLDC_02_controller_v3_1_work1/mode set logic ==
  state set_actual_mode
    state set_autonomous_targets
      en: armed_flag = true;
      en: operation_mode = uint8(1);
    state swich_off_if_high_pitch
      en: operation_mode = uint8(0);
    (default) -> (junction 22)
    (junction 22) -> swich_off_if_high_pitch [order 1] : [abs(pitch_actual)>50*2*pi/360]
    (junction 22) -> set_autonomous_targets [order 2]
    swich_off_if_high_pitch -> set_actual_mode
    set_autonomous_targets -> set_actual_mode
  (default) -> set_actual_mode
  data: armed_flag output boolean size=1; operation_mode output uint8 size=1; pitch_actual input double size=1
  events: t_fc_mode_set_logic input FUNCTION_CALL_EVENT

== stateflow chart MECROKA_TWR_BLDC_02_controller_v3_1_work1/autonomous targets ==
  state set_autonomous_targets
    state Op_mode_fast_mode
      state stop2
        en, du: vel_trgt_auto   = 0.00;
        en, du: yaw_rate_trgt_auto  = 0.0;
      state stop1
        en, du: vel_trgt_auto   = 0.00;
        en, du: yaw_rate_trgt_auto  = 0.0;
        en, du: Position_target= 0.0;
      state Go
        en, du: vel_trgt_auto  = 01;
        en, du: yaw_rate_trgt_auto  = 0.0;
        en, du: Position_target= 3.1;
      state stop4
        en, du: vel_trgt_auto   = 0.0;
        en, du: yaw_rate_trgt_auto  = 0.0;
        en, du: Position_target= 3;
      state stop3
        en, du: vel_trgt_auto   = 0.0;
        en, du: yaw_rate_trgt_auto  = 0.0;
        en, du: Position_target= 3.1;
      (default) -> set_autonomous_targets.Op_mode_fast_mode.stop1
      set_autonomous_targets.Op_mode_fast_mode.stop1 -> set_autonomous_targets.Op_mode_fast_mode.Go : [after(5,sec)]
      set_autonomous_targets.Op_mode_fast_mode.stop4 -> set_autonomous_targets.Op_mode_fast_mode.stop2 : [after(5,sec)]
      set_autonomous_targets.Op_mode_fast_mode.Go -> set_autonomous_targets.Op_mode_fast_mode.stop3 : [after(1.5,sec)]
      set_autonomous_targets.Op_mode_fast_mode.stop3 -> set_autonomous_targets.Op_mode_fast_mode.stop4 : [after(3,sec)]
    state OP_mode_stop_and_go_3
      state stop1
        en, du: vel_trgt_auto   = 0.00;
        en, du: yaw_rate_trgt_auto  = 0.0;
      state turn
        en, du: vel_trgt_auto   = 0.0;
        en, du: yaw_rate_trgt_auto  = pi/2;
      state stop2
        en, du: vel_trgt_auto   = 0.00;
        en, du: yaw_rate_trgt_auto  = 0.0;
      state go_forward
        en, du: vel_trgt_auto   = 0.4;
        en, du: yaw_rate_trgt_auto  = 0.0;
      (default) -> set_autonomous_targets.OP_mode_stop_and_go_3.stop1
      set_autonomous_targets.OP_mode_stop_and_go_3.stop1 -> turn : after(5,sec)
      turn -> set_autonomous_targets.OP_mode_stop_and_go_3.stop2 : after(1,sec)
      set_autonomous_targets.OP_mode_stop_and_go_3.stop2 -> go_forward : after(5,sec)
      go_forward -> OP_mode_stop_and_go_3 : after(5,sec)
    state Op_mode_pattern_8
      state stop2
        en, du: vel_trgt_auto   = 0.00;
        en, du: yaw_rate_trgt_auto  = 0.0;
      state stop1
        en, du: vel_trgt_auto   = 0.00;
        en, du: yaw_rate_trgt_auto  = 0.0;
      state Go
        en, du: vel_trgt_auto   = 0.8;
        en, du: yaw_rate_trgt_auto  = 0.0;
      state stop3
        en, du: vel_trgt_auto   = 0.8;
        en, du: yaw_rate_trgt_auto  = pi/1.96;
      state stop5
        en, du: vel_trgt_auto   = 0.8;
        en, du: yaw_rate_trgt_auto  = pi/1.96;
      state stop4
        en, du: vel_trgt_auto   = 0.8;
        en, du: yaw_rate_trgt_auto  = -pi/1.96;
      (default) -> set_autonomous_targets.Op_mode_pattern_8.stop1
      set_autonomous_targets.Op_mode_pattern_8.stop1 -> set_autonomous_targets.Op_mode_pattern_8.Go : [after(5,sec)]
      stop5 -> set_autonomous_targets.Op_mode_pattern_8.stop2 : [after(2,sec)]
      set_autonomous_targets.Op_mode_pattern_8.Go -> set_autonomous_targets.Op_mode_pattern_8.stop3 : [after(3,sec)]
      set_autonomous_targets.Op_mode_pattern_8.stop3 -> set_autonomous_targets.Op_mode_pattern_8.stop4 : [after(2,sec)]
      set_autonomous_targets.Op_mode_pattern_8.stop4 -> stop5 : [after(4,sec)]
    state Op_mode_steady_balancing_1
      state stop1
        en, du: vel_trgt_auto   = 0.00;
        en, du: yaw_rate_trgt_auto  = 0.0;
        en, du: Position_target= 0.0;
      state stop2
        en, du: vel_trgt_auto   = 0.00;
        en, du: yaw_rate_trgt_auto  = 0.0;
      state Go
        en, du: vel_trgt_auto  = 01;
        en, du: yaw_rate_trgt_auto  = 0.0;
        en, du: Position_target= 3;
      state stop3
        en, du: vel_trgt_auto   = 0.0;
        en, du: yaw_rate_trgt_auto  = 0.0;
        en, du: Position_target= 3;
      (default) -> set_autonomous_targets.Op_mode_steady_balancing_1.stop1
      set_autonomous_targets.Op_mode_steady_balancing_1.stop1 -> set_autonomous_targets.Op_mode_steady_balancing_1.Go : [after(5,sec)]
      set_autonomous_targets.Op_mode_steady_balancing_1.stop3 -> set_autonomous_targets.Op_mode_steady_balancing_1.stop2 : [after(10,sec)]
      set_autonomous_targets.Op_mode_steady_balancing_1.Go -> set_autonomous_targets.Op_mode_steady_balancing_1.stop3 : [after(10,sec)]
    state OP_mode_off_0
      en, du: vel_trgt_auto   = 0.00;
      en, du: yaw_rate_trgt_auto  = 0.0;
    (default) -> (junction 57)
    (junction 57) -> Op_mode_fast_mode [order 1] : [op_mode == 1 ]
    (junction 57) -> (junction 59) [order 2]
    (junction 59) -> (junction 58)
    (junction 58) -> Op_mode_pattern_8 [order 1] : [op_mode == 5]
    (junction 58) -> (junction 61) [order 2]
    (junction 61) -> OP_mode_stop_and_go_3 [order 1] : [op_mode == 3]
    (junction 61) -> (junction 62) [order 2]
    (junction 62) -> Op_mode_steady_balancing_1 [order 1] : [op_mode == 6 ]
    (junction 62) -> OP_mode_off_0 [order 2]
  (default) -> set_autonomous_targets
  data: op_mode input uint8 size=1; vel_trgt_auto output double size=1; yaw_rate_trgt_auto output double size=1; Position_target output double
  events: t_fc_auto_trgts input FUNCTION_CALL_EVENT
